simulink model "project_1"  (R2023a)
settings: Solver=FixedStepDiscrete  StartTime=0.0  StopTime=inf  FixedStep=0.01  RelTol=1e-3  EnableMultiTasking=on
libraries: arduinolib x9, arduinosensorlib x1
settings Model: ExtModeTrigDuration=2  Creator=admin  LastModifiedBy=admin
settings OptimizationCC: EnhancedBackFolding=on  PassReuseOutputArgsAs=Individual arguments  ZeroExternalMemoryAtStartup=off  ZeroInternalMemoryAtStartup=off  MaxStackSize=64  OptimizeBlockOrder=speed  DifferentSizesBufferReuse=on  OptimizationCustomize=off  EfficientTunableParamExpr=on
settings DebuggingCC: ParameterTunabilityLossMsg=error
settings HardwareCC: ProdBitPerInt=16  ProdBitPerPointer=16  ProdBitPerSizeT=16  ProdBitPerPtrDiffT=16  ProdLargestAtomicFloat=None  ProdWordSize=8  ProdHWDeviceType=Atmel->AVR
settings SFSimCC: MATLABDynamicMemAlloc=off
settings RTWCC: Description=Embedded Coder  SystemTargetFile=ert.tlc  HardwareBoard=Arduino Mega 2560  TemplateMakefile=ert_default_tmf  Toolchain=Arduino AVR  BuildConfiguration=Faster Runs
settings CodeAppCC: ForceParamTrailComments=on  IgnoreCustomStorageClasses=off  OperatorAnnotations=on  SimulinkDataObjDesc=on  SFDataObjDesc=on  InsertBlockDesc=on
settings ERTTargetCC: SupportContinuousTime=on  SupportVariableSizeSignals=on  ExtModeTransport=3  ExtModeStaticAlloc=on  ExtModeAutomaticAllocSize=off  ExtModeStaticAllocSize=2048  ExtModeMexFile=ext_xcp  ExtModeIntrfLevel=Level2 - Open

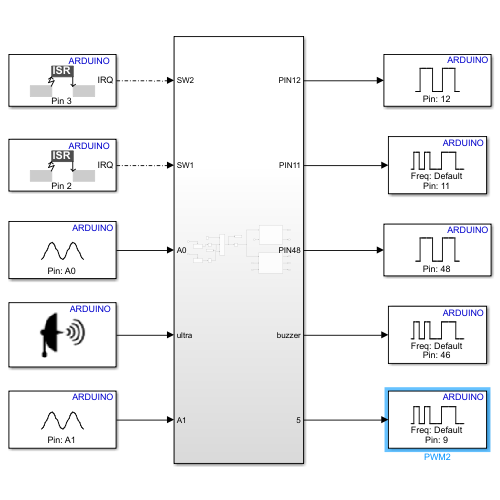
[thumbnail: Simulink's stored preview of the top-level diagram]
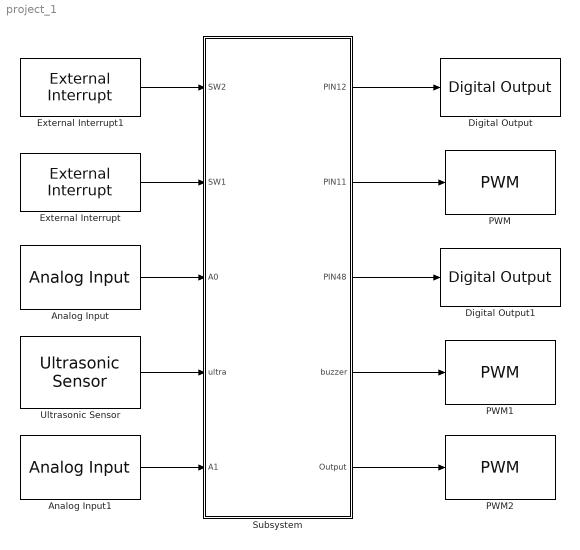
== system project_1 ==
  Analog Input : arduinolib/Analog Input  pinNumber=0  ReadResultsOnly=off  ConversionTriggerSource=Software  ExternalTriggerType=uint32( 0 )  OutputDataType=uint16  EnableConversionCompleteNotify=off  EnableOuputStatus=off  SampleTime=-1  blockPlatform=arduino
  Analog Input1 : arduinolib/Analog Input  pinNumber=1  ReadResultsOnly=off  ConversionTriggerSource=Software  ExternalTriggerType=uint32( 0 )  OutputDataType=uint16  EnableConversionCompleteNotify=off  EnableOuputStatus=off  SampleTime=-1  blockPlatform=arduino
  Digital Output : arduinolib/Digital Output  pinNumber=12  Direction=output  blockPlatform=arduino
  Digital Output1 : arduinolib/Digital Output  pinNumber=48  Direction=output  blockPlatform=arduino
  External Interrupt : arduinolib/External Interrupt  Pin=2  PullUp=off  Mode=FALLING  InterruptSimulationInput=off
  External Interrupt1 : arduinolib/External Interrupt  Pin=3  PullUp=off  Mode=FALLING  InterruptSimulationInput=off
  PWM : arduinolib/PWM  pinNumber=11  frequencyType=Default  desiredFrequency=490.2  achievableFrequency=490.2
  PWM1 : arduinolib/PWM  pinNumber=46  frequencyType=Default  desiredFrequency=490.2  achievableFrequency=490.2
  PWM2 : arduinolib/PWM  pinNumber=9  frequencyType=Default  desiredFrequency=490.2  achievableFrequency=490.2
  Subsystem : Subsystem
  Ultrasonic Sensor : arduinosensorlib/Ultrasonic Sensor  NumSignalPins=2  TrigPin=50  EchoPin=51  SignalPin=3  SampleTime_=0.1  blockPlatform=ARDUINO
  wires:
  External Interrupt1/1 -> Subsystem/1(SW2)
  External Interrupt/1 -> Subsystem/2(SW1)
  Subsystem/1(PIN12) -> Digital Output/1
  Subsystem/2(PIN11) -> PWM/1
  Analog Input/1 -> Subsystem/3(A0)
  Subsystem/3(PIN48) -> Digital Output1/1
  Ultrasonic Sensor/1 -> Subsystem/4(ultra)
  Subsystem/4(buzzer) -> PWM1/1
  Analog Input1/1 -> Subsystem/5(A1)
  Subsystem/5(Output) -> PWM2/1

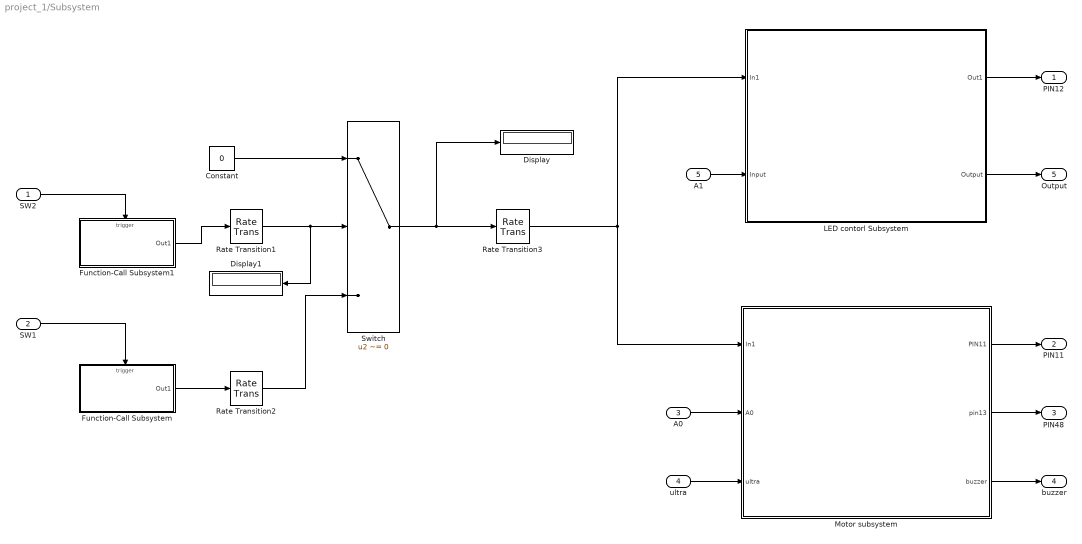
== system project_1/Subsystem ==
  SW2 : Inport
  SW1 : Inport  Port=2
  A0 : Inport  Port=3
  ultra : Inport  Port=4
  A1 : Inport  Port=5
  Constant : Constant  Value=0
  Display : Display
  Display1 : Display
  Function-Call Subsystem : Subsystem  TreatAsAtomicUnit=on
  Function-Call Subsystem1 : Subsystem  TreatAsAtomicUnit=on
  LED contorl Subsystem : Subsystem
  Motor subsystem : Subsystem
  Rate Transition1 : RateTransition  Deterministic=off
  Rate Transition2 : RateTransition  Deterministic=off
  Rate Transition3 : RateTransition  Deterministic=off
  Switch : Switch  Criteria=u2 ~= 0  SaturateOnIntegerOverflow=off  InputSameDT=off
  PIN12 : Outport
  PIN11 : Outport  Port=2
  PIN48 : Outport  Port=3
  buzzer : Outport  Port=4
  Output : Outport  Port=5
  wires:
  SW2/1 -> Function-Call Subsystem1/Trigger
  Function-Call Subsystem1/1(Out1) -> Rate Transition1/1
  Switch/1 -> Rate Transition3/1, Display/1
  Rate Transition3/1 -> Motor subsystem/1(In1), LED contorl Subsystem/1(In1)
  Rate Transition1/1 -> Display1/1, Switch/2
  Constant/1 -> Switch/1
  Rate Transition2/1 -> Switch/3
  Function-Call Subsystem/1(Out1) -> Rate Transition2/1
  SW1/1 -> Function-Call Subsystem/Trigger
  LED contorl Subsystem/1(Out1) -> PIN12/1
  A0/1 -> Motor subsystem/2(A0)
  Motor subsystem/1(PIN11) -> PIN11/1
  ultra/1 -> Motor subsystem/3(ultra)
  Motor subsystem/2(pin13) -> PIN48/1
  Motor subsystem/3(buzzer) -> buzzer/1
  A1/1 -> LED contorl Subsystem/2(Input)
  LED contorl Subsystem/2(Output) -> Output/1

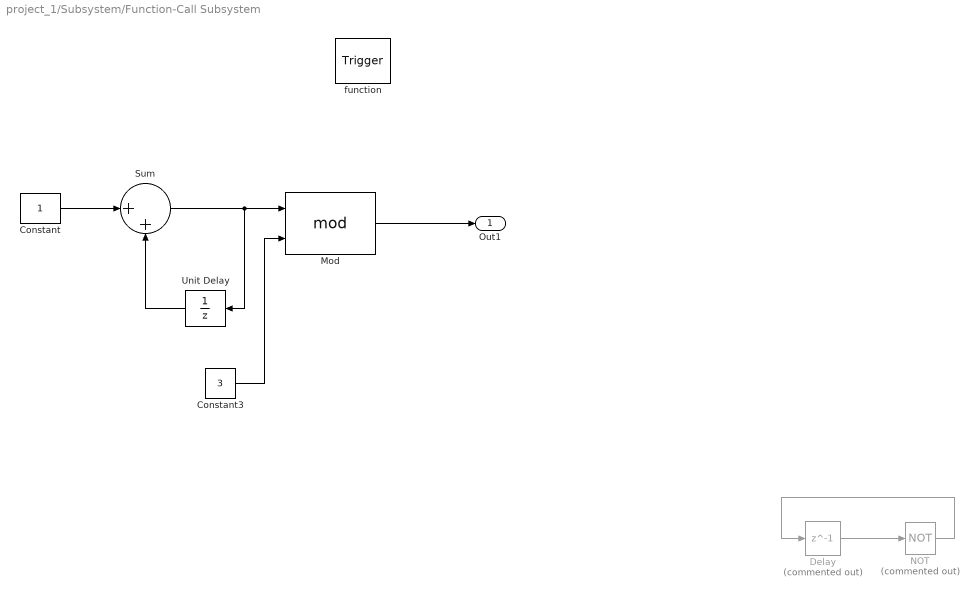
== system project_1/Subsystem/Function-Call Subsystem ==
  function : TriggerPort  TriggerType=function-call  VariantControl=(inherit)
  Constant : Constant
  Constant3 : Constant  Value=3
  Delay : Delay  Commented=on  DelayLength=1  InitialCondition=0
  Mod : Math  Operator=mod
  NOT : Logic  Commented=on  Operator=NOT  IconShape=distinctive  AllPortsSameDT=off  OutDataTypeStr=boolean
  Sum : Sum  Inputs=|++
  Unit Delay : UnitDelay  SampleTime=-1  HasFrameUpgradeWarning=on
  Out1 : Outport
  wires:
  Constant/1 -> Sum/1
  Unit Delay/1 -> Sum/2
  Constant3/1 -> Mod/2
  Sum/1 -> Unit Delay/1, Mod/1
  NOT/1 -> Delay/1
  Delay/1 -> NOT/1
  Mod/1 -> Out1/1

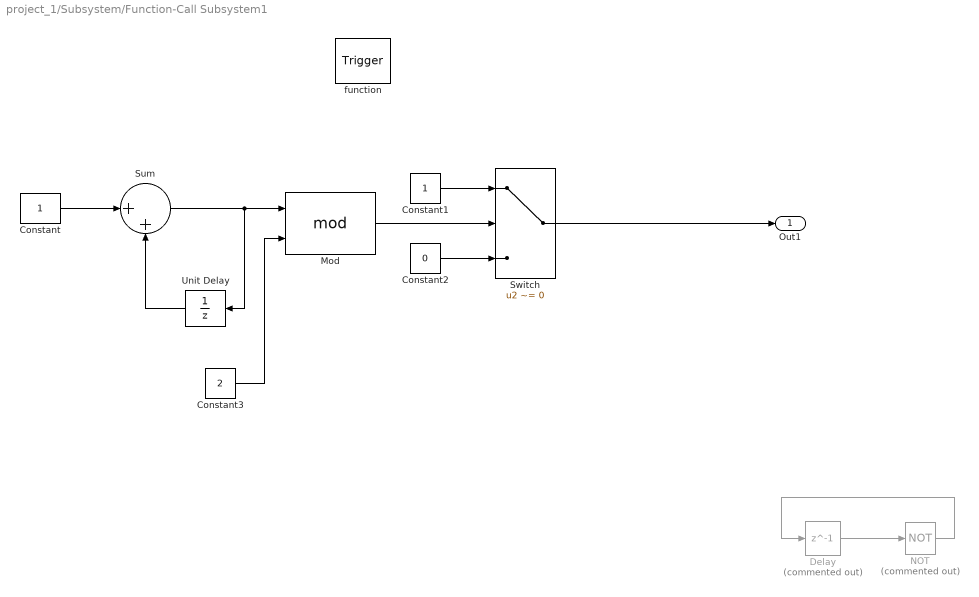
== system project_1/Subsystem/Function-Call Subsystem1 ==
  function : TriggerPort  TriggerType=function-call  VariantControl=(inherit)
  Constant : Constant
  Constant1 : Constant
  Constant2 : Constant  Value=0
  Constant3 : Constant  Value=2
  Delay : Delay  Commented=on  DelayLength=1  InitialCondition=0
  Mod : Math  Operator=mod
  NOT : Logic  Commented=on  Operator=NOT  IconShape=distinctive  AllPortsSameDT=off  OutDataTypeStr=boolean
  Sum : Sum  Inputs=|++
  Switch : Switch  Criteria=u2 ~= 0  SaturateOnIntegerOverflow=off  InputSameDT=off
  Unit Delay : UnitDelay  SampleTime=-1  HasFrameUpgradeWarning=on
  Out1 : Outport
  wires:
  Delay/1 -> NOT/1
  NOT/1 -> Delay/1
  Mod/1 -> Switch/2
  Sum/1 -> Mod/1, Unit Delay/1
  Constant3/1 -> Mod/2
  Constant2/1 -> Switch/3
  Constant1/1 -> Switch/1
  Unit Delay/1 -> Sum/2
  Switch/1 -> Out1/1
  Constant/1 -> Sum/1

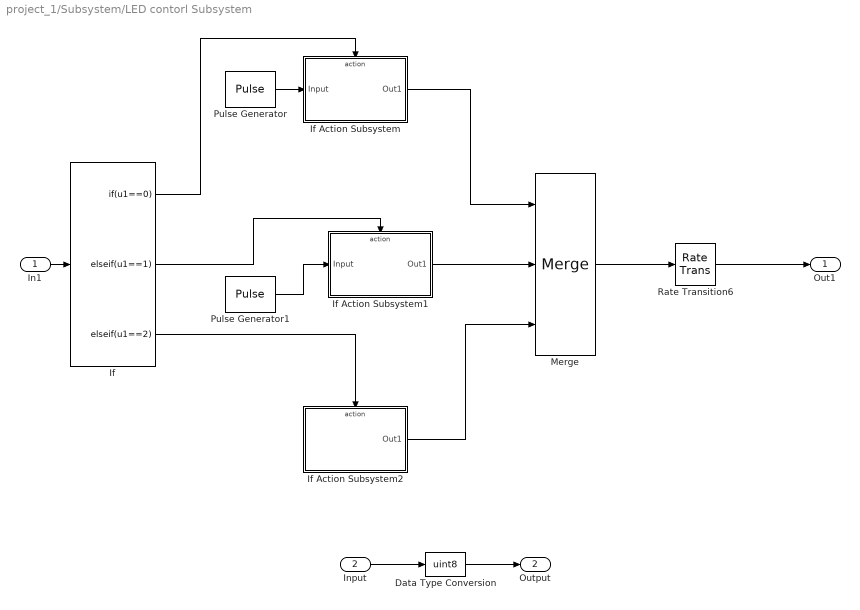
== system project_1/Subsystem/LED contorl Subsystem ==
  In1 : Inport
  Input : Inport  Port=2
  Data Type Conversion : DataTypeConversion  OutDataTypeStr=uint8  SaturateOnIntegerOverflow=off  RndMeth=Floor
  If : If  IfExpression=u1==0  ElseIfExpressions=u1==1,u1==2  ShowElse=off
  If Action Subsystem : Subsystem  TreatAsAtomicUnit=on
  If Action Subsystem1 : Subsystem  TreatAsAtomicUnit=on
  If Action Subsystem2 : Subsystem  TreatAsAtomicUnit=on
  Merge : Merge  Inputs=3
  Pulse Generator : DiscretePulseGenerator  PulseType=Time based  PulseWidth=50
  Pulse Generator1 : DiscretePulseGenerator  PulseType=Time based  Period=0.4  PulseWidth=50
  Rate Transition6 : RateTransition  Deterministic=off
  Out1 : Outport
  Output : Outport  Port=2
  wires:
  If/3 -> If Action Subsystem2/Action
  If Action Subsystem2/1(Out1) -> Merge/3
  If/1 -> If Action Subsystem/Action
  If/2 -> If Action Subsystem1/Action
  Pulse Generator/1 -> If Action Subsystem/1(Input)
  If Action Subsystem1/1(Out1) -> Merge/2
  Pulse Generator1/1 -> If Action Subsystem1/1(Input)
  If Action Subsystem/1(Out1) -> Merge/1
  Merge/1 -> Rate Transition6/1
  In1/1 -> If/1
  Rate Transition6/1 -> Out1/1
  Data Type Conversion/1 -> Output/1
  Input/1 -> Data Type Conversion/1

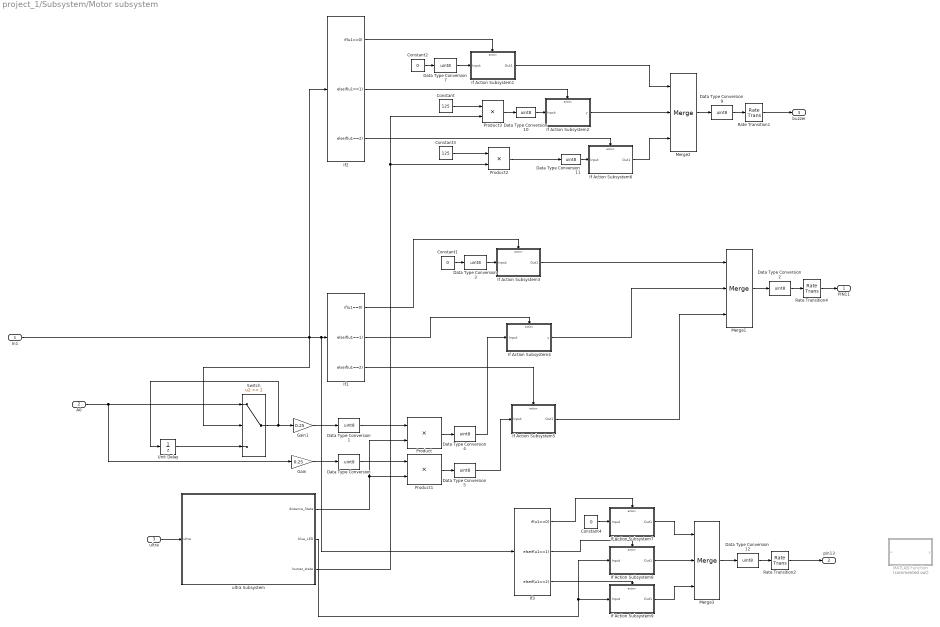
== system project_1/Subsystem/Motor subsystem ==
  In1 : Inport
  A0 : Inport  Port=2
  ultra : Inport  Port=3
  Constant : Constant  Value=125
  Constant1 : Constant  Value=0
  Constant2 : Constant  Value=0
  Constant3 : Constant  Value=125
  Constant4 : Constant  Value=0
  Data Type Conversion{,1..5,7,9..12} (11 alike) : DataTypeConversion  OutDataTypeStr=uint8  SaturateOnIntegerOverflow=off  RndMeth=Floor
  Gain : Gain  Gain=0.25
  Gain1 : Gain  Gain=0.25
  If Action Subsystem1 : Subsystem  TreatAsAtomicUnit=on
  If Action Subsystem2 : Subsystem  TreatAsAtomicUnit=on
  If Action Subsystem3 : Subsystem  TreatAsAtomicUnit=on
  If Action Subsystem4 : Subsystem  TreatAsAtomicUnit=on
  If Action Subsystem5 : Subsystem  TreatAsAtomicUnit=on
  If Action Subsystem6 : Subsystem  TreatAsAtomicUnit=on
  If Action Subsystem7 : Subsystem  TreatAsAtomicUnit=on
  If Action Subsystem8 : Subsystem  TreatAsAtomicUnit=on
  If Action Subsystem9 : Subsystem  TreatAsAtomicUnit=on
  If1 : If  IfExpression=u1==0  ElseIfExpressions=u1==1,u1==2  ShowElse=off
  If2 : If  IfExpression=u1==0  ElseIfExpressions=u1==1,u1==2  ShowElse=off
  If3 : If  IfExpression=u1==0  ElseIfExpressions=u1==1,u1==2  ShowElse=off
  MATLAB Function : MATLAB Function  Commented=on  TreatAsAtomicUnit=on
  Merge1 : Merge  Inputs=3
  Merge2 : Merge  Inputs=3
  Merge3 : Merge  Inputs=3
  Product : Product
  Product1 : Product
  Product2 : Product  OutDataTypeStr=double
  Product3 : Product  OutDataTypeStr=double
  Rate Transition1 : RateTransition  Deterministic=off
  Rate Transition2 : RateTransition  Deterministic=off
  Rate Transition4 : RateTransition  Deterministic=off
  Switch : Switch  Threshold=2  SaturateOnIntegerOverflow=off  InputSameDT=off
  Unit Delay : UnitDelay  SampleTime=-1  HasFrameUpgradeWarning=on
  ultra Subsystem : Subsystem
  PIN11 : Outport
  pin13 : Outport  Port=2
  buzzer : Outport  Port=3
  wires:
  A0/1 -> Switch/1, Gain/1
  If1/3 -> If Action Subsystem5/Action
  Constant1/1 -> Data Type Conversion3/1
  If1/2 -> If Action Subsystem4/Action
  Data Type Conversion2/1 -> Rate Transition4/1
  Gain1/1 -> Data Type Conversion1/1
  Gain/1 -> Data Type Conversion/1
  If1/1 -> If Action Subsystem3/Action
  Data Type Conversion3/1 -> If Action Subsystem3/1(Input)
  If Action Subsystem3/1(Out1) -> Merge1/1
  Rate Transition4/1 -> PIN11/1
  Merge1/1 -> Data Type Conversion2/1
  In1/1 -> If1/1, If3/1, If2/1, Switch/2
  If Action Subsystem4/1(y) -> Merge1/2
  If Action Subsystem5/1(Out1) -> Merge1/3
  Product/1 -> Data Type Conversion4/1
  Data Type Conversion4/1 -> If Action Subsystem4/1(Input)
  Product1/1 -> Data Type Conversion5/1
  Data Type Conversion5/1 -> If Action Subsystem5/1(Input)
  Data Type Conversion/1 -> Product1/1
  Data Type Conversion1/1 -> Product/1
  ultra/1 -> ultra Subsystem/1(ultra)
  ultra Subsystem/1(distance_State) -> Product/2, Product1/2
  Switch/1 -> Unit Delay/1, Gain1/1
  Unit Delay/1 -> Switch/3
  If2/1 -> If Action Subsystem1/Action
  Constant2/1 -> Data Type Conversion7/1
  Data Type Conversion7/1 -> If Action Subsystem1/1(Input)
  If2/2 -> If Action Subsystem2/Action
  If2/3 -> If Action Subsystem6/Action
  If Action Subsystem1/1(Out1) -> Merge2/1
  If Action Subsystem2/1(y) -> Merge2/2
  If Action Subsystem6/1(Out1) -> Merge2/3
  Data Type Conversion9/1 -> Rate Transition1/1
  Merge2/1 -> Data Type Conversion9/1
  ultra Subsystem/3(buzzer_state) -> Product2/2, Product3/2
  Data Type Conversion10/1 -> If Action Subsystem2/1(Input)
  Product3/1 -> Data Type Conversion10/1
  Product2/1 -> Data Type Conversion11/1
  Data Type Conversion11/1 -> If Action Subsystem6/1(Input)
  If3/1 -> If Action Subsystem7/Action
  If3/2 -> If Action Subsystem8/Action
  If3/3 -> If Action Subsystem9/Action
  Constant4/1 -> If Action Subsystem7/1(Input)
  Merge3/1 -> Data Type Conversion12/1
  Data Type Conversion12/1 -> Rate Transition2/1
  Rate Transition2/1 -> pin13/1
  If Action Subsystem7/1(Out1) -> Merge3/1
  If Action Subsystem8/1(Out1) -> Merge3/2
  If Action Subsystem9/1(Out1) -> Merge3/3
  ultra Subsystem/2(blue_LED) -> If Action Subsystem9/1(Input), If Action Subsystem8/1(Input)
  Rate Transition1/1 -> buzzer/1
  Constant/1 -> Product3/1
  Constant3/1 -> Product2/1

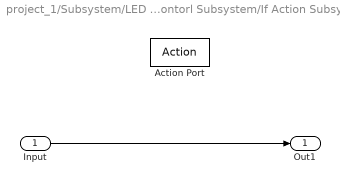
== system project_1/Subsystem/LED contorl Subsystem/If Action Subsystem ==
  Input : Inport
  Action Port : ActionPort  ActionPortLabel=if(u1==0)
  Out1 : Outport
  wires:
  Input/1 -> Out1/1

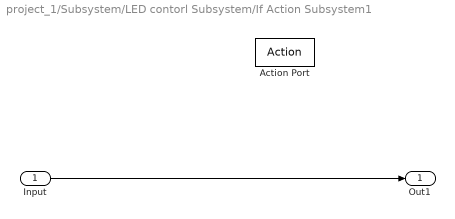
== system project_1/Subsystem/LED contorl Subsystem/If Action Subsystem1 ==
  Input : Inport
  Action Port : ActionPort  ActionPortLabel=elseif(u1==1)
  Out1 : Outport
  wires:
  Input/1 -> Out1/1

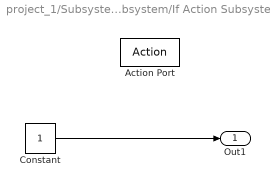
== system project_1/Subsystem/LED contorl Subsystem/If Action Subsystem2 ==
  Action Port : ActionPort  ActionPortLabel=elseif(u1==2)
  Constant : Constant
  Out1 : Outport
  wires:
  Constant/1 -> Out1/1

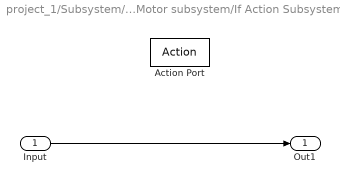
== system project_1/Subsystem/Motor subsystem/If Action Subsystem1 ==
  Input : Inport
  Action Port : ActionPort  ActionPortLabel=if(u1==0)
  Out1 : Outport
  wires:
  Input/1 -> Out1/1

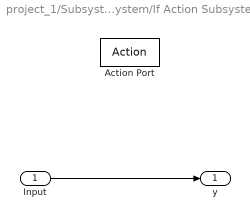
== system project_1/Subsystem/Motor subsystem/If Action Subsystem2 ==
  Input : Inport
  Action Port : ActionPort  ActionPortLabel=elseif(u1==1)
  y : Outport
  wires:
  Input/1 -> y/1

== system project_1/Subsystem/Motor subsystem/If Action Subsystem3 ==
  Input : Inport
  Action Port : ActionPort  ActionPortLabel=if(u1==0)
  Out1 : Outport
  wires:
  Input/1 -> Out1/1

== system project_1/Subsystem/Motor subsystem/If Action Subsystem4 ==
  Input : Inport
  Action Port : ActionPort  ActionPortLabel=elseif(u1==1)
  y : Outport
  wires:
  Input/1 -> y/1

== system project_1/Subsystem/Motor subsystem/If Action Subsystem5 ==
  Input : Inport
  Action Port : ActionPort  ActionPortLabel=elseif(u1==2)
  Out1 : Outport
  wires:
  Input/1 -> Out1/1

== system project_1/Subsystem/Motor subsystem/If Action Subsystem6 ==
  Input : Inport
  Action Port : ActionPort  ActionPortLabel=elseif(u1==2)
  Out1 : Outport
  wires:
  Input/1 -> Out1/1

== system project_1/Subsystem/Motor subsystem/If Action Subsystem7 ==
  Input : Inport
  Action Port : ActionPort  ActionPortLabel=if(u1==0)
  Out1 : Outport
  wires:
  Input/1 -> Out1/1

== system project_1/Subsystem/Motor subsystem/If Action Subsystem8 ==
  Input : Inport
  Action Port : ActionPort  ActionPortLabel=elseif(u1==1)
  Out1 : Outport
  wires:
  Input/1 -> Out1/1

== system project_1/Subsystem/Motor subsystem/If Action Subsystem9 ==
  Input : Inport
  Action Port : ActionPort  ActionPortLabel=elseif(u1==2)
  Out1 : Outport
  wires:
  Input/1 -> Out1/1

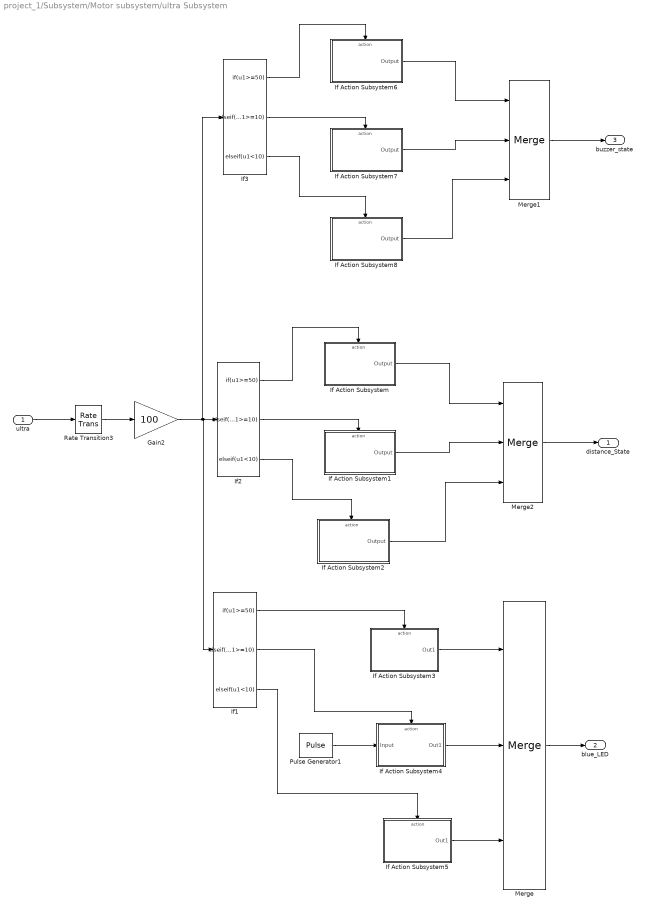
== system project_1/Subsystem/Motor subsystem/ultra Subsystem ==
  ultra : Inport
  Gain2 : Gain  Gain=100
  If Action Subsystem : Subsystem  TreatAsAtomicUnit=on
  If Action Subsystem1 : Subsystem  TreatAsAtomicUnit=on
  If Action Subsystem2 : Subsystem  TreatAsAtomicUnit=on
  If Action Subsystem3 : Subsystem  TreatAsAtomicUnit=on
  If Action Subsystem4 : Subsystem  TreatAsAtomicUnit=on
  If Action Subsystem5 : Subsystem  TreatAsAtomicUnit=on
  If Action Subsystem6 : Subsystem  TreatAsAtomicUnit=on
  If Action Subsystem7 : Subsystem  TreatAsAtomicUnit=on
  If Action Subsystem8 : Subsystem  TreatAsAtomicUnit=on
  If1 : If  IfExpression=u1>=50  ElseIfExpressions=u1<50 & u1>=10, u1<10  ShowElse=off
  If2 : If  IfExpression=u1>=50  ElseIfExpressions=u1<50 & u1>=10, u1<10  ShowElse=off
  If3 : If  IfExpression=u1>=50  ElseIfExpressions=u1<50 & u1>=10, u1<10  ShowElse=off
  Merge : Merge  Inputs=3
  Merge1 : Merge  Inputs=3
  Merge2 : Merge  Inputs=3
  Pulse Generator1 : DiscretePulseGenerator  PulseType=Time based  Period=0.4  PulseWidth=50
  Rate Transition3 : RateTransition  Deterministic=off
  distance_State : Outport
  blue_LED : Outport  Port=2
  buzzer_state : Outport  Port=3
  wires:
  Rate Transition3/1 -> Gain2/1
  If2/1 -> If Action Subsystem/Action
  If2/3 -> If Action Subsystem2/Action
  Gain2/1 -> If3/1, If1/1, If2/1
  If2/2 -> If Action Subsystem1/Action
  Merge2/1 -> distance_State/1
  Pulse Generator1/1 -> If Action Subsystem4/1(Input)
  If Action Subsystem5/1(Out1) -> Merge/3
  If Action Subsystem4/1(Out1) -> Merge/2
  If1/1 -> If Action Subsystem3/Action
  If Action Subsystem3/1(Out1) -> Merge/1
  If1/2 -> If Action Subsystem4/Action
  If1/3 -> If Action Subsystem5/Action
  ultra/1 -> Rate Transition3/1
  If Action Subsystem/1(Output) -> Merge2/1
  If Action Subsystem1/1(Output) -> Merge2/2
  If Action Subsystem2/1(Output) -> Merge2/3
  Merge/1 -> blue_LED/1
  If Action Subsystem8/1(Output) -> Merge1/3
  If Action Subsystem6/1(Output) -> Merge1/1
  If3/1 -> If Action Subsystem6/Action
  If3/2 -> If Action Subsystem7/Action
  If Action Subsystem7/1(Output) -> Merge1/2
  If3/3 -> If Action Subsystem8/Action
  Merge1/1 -> buzzer_state/1

== system project_1/Subsystem/Motor subsystem/ultra Subsystem/If Action Subsystem ==
  Action Port : ActionPort  ActionPortLabel=if(u1>=50)
  Constant : Constant
  Output : Outport
  wires:
  Constant/1 -> Output/1

== system project_1/Subsystem/Motor subsystem/ultra Subsystem/If Action Subsystem1 ==
  Action Port : ActionPort  ActionPortLabel=elseif(u1<50 & u1>=10)
  Constant : Constant  Value=0.5
  Output : Outport
  wires:
  Constant/1 -> Output/1

== system project_1/Subsystem/Motor subsystem/ultra Subsystem/If Action Subsystem2 ==
  Action Port : ActionPort  ActionPortLabel=elseif( u1<10)
  Constant : Constant  Value=0
  Output : Outport
  wires:
  Constant/1 -> Output/1

== system project_1/Subsystem/Motor subsystem/ultra Subsystem/If Action Subsystem3 ==
  Action Port : ActionPort  ActionPortLabel=if(u1>=50)
  Constant : Constant  Value=0
  Out1 : Outport
  wires:
  Constant/1 -> Out1/1

== system project_1/Subsystem/Motor subsystem/ultra Subsystem/If Action Subsystem4 ==
  Input : Inport
  Action Port : ActionPort  ActionPortLabel=elseif(u1<50 & u1>=10)
  Out1 : Outport
  wires:
  Input/1 -> Out1/1

== system project_1/Subsystem/Motor subsystem/ultra Subsystem/If Action Subsystem5 ==
  Action Port : ActionPort  ActionPortLabel=elseif( u1<10)
  Constant : Constant
  Out1 : Outport
  wires:
  Constant/1 -> Out1/1

== system project_1/Subsystem/Motor subsystem/ultra Subsystem/If Action Subsystem6 ==
  Action Port : ActionPort  ActionPortLabel=if(u1>=50)
  Constant : Constant  Value=0
  Output : Outport
  wires:
  Constant/1 -> Output/1

== system project_1/Subsystem/Motor subsystem/ultra Subsystem/If Action Subsystem7 ==
  Action Port : ActionPort  ActionPortLabel=elseif(u1<50 & u1>=10)
  Constant : Constant  Value=0.5
  Output : Outport
  wires:
  Constant/1 -> Output/1

== system project_1/Subsystem/Motor subsystem/ultra Subsystem/If Action Subsystem8 ==
  Action Port : ActionPort  ActionPortLabel=elseif( u1<10)
  Constant : Constant  Value=2
  Output : Outport
  wires:
  Constant/1 -> Output/1

== matlab function project_1/Subsystem/Motor subsystem/MATLAB Function ==
  data: u input; y output
function y = fcn(u)
persistent fixed;
persistent flag;

if isempty(flag)
    fixed = u;
    flag = false;
end


y = fixed
